simulink model "ILC_Intro"  (R2019a)
settings: Solver=VariableStepAuto  StartTime=0.0  StopTime=10.0  RelTol=1e-3
undefined symbols (not defined in the file or in its folder): K
libraries: cstblocks x1
settings Model: Creator=capn  LastModifiedBy=emma
settings DataIOCC: ReturnWorkspaceOutputs=off
settings DebuggingCC: ArithmeticOperatorsInVariantConditions=warning
settings SFSimCC: SimUseLocalCustomCode=off
settings RTWCC: RTWUseLocalCustomCode=off
settings CodeAppCC: StateflowObjectComments=on

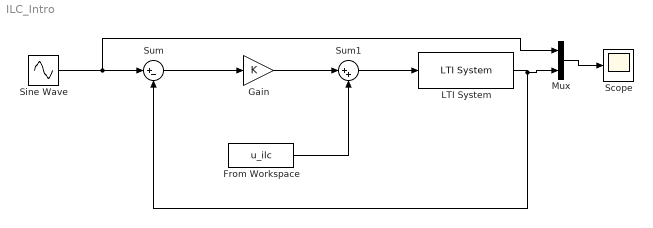
== system ILC_Intro ==
  From Workspace : FromWorkspace  VariableName=u_ilc  SampleTime=0
  Gain : Gain  Gain=K
  LTI System : cstblocks/LTI System  sys=Pd  IC=[]
  Mux : Mux  Inputs=2
  Scope : Scope
  Sine Wave : Sin  SampleTime=0
  Sum : Sum  Inputs=|+-
  Sum1 : Sum  Inputs=|++
  wires:
  Sum/1 -> Gain/1
  Gain/1 -> Sum1/1
  Sum1/1 -> LTI System/1
  Sine Wave/1 -> Mux/1, Sum/1
  From Workspace/1 -> Sum1/2
  LTI System/1 -> Mux/2, Sum/2
  Mux/1 -> Scope/1
